simulink model "Buck_Converter_Model"  (R2020a)
settings: Solver=VariableStepAuto  StartTime=0.0  StopTime=0.4  RelTol=1e-3
libraries: powerlib x16, powerlib_meascontrol x2
settings Model: Creator=Ricardo Romero  LastModifiedBy=Ricardo Romero

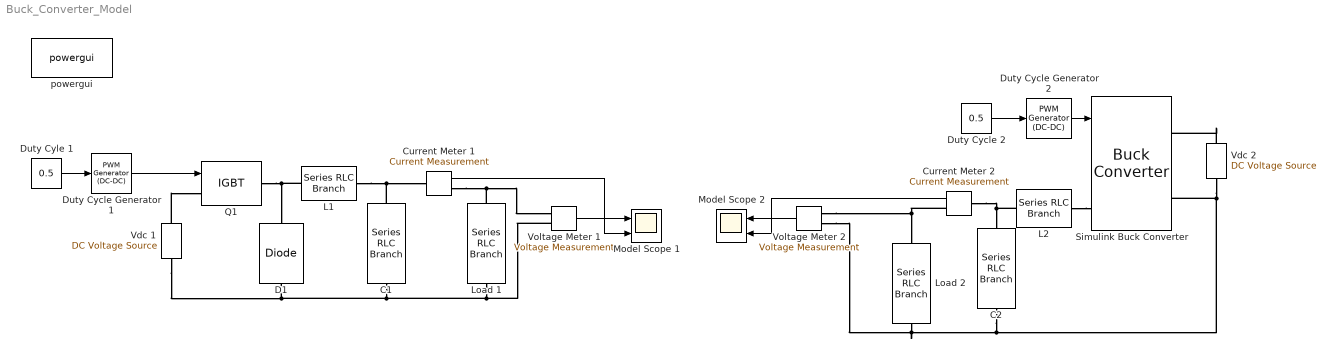
== system Buck_Converter_Model ==
  C1 : powerlib/Elements/Series RLC Branch  LConnTagsString=__new0  RConnTagsString=__new0  BranchType=C  Resistance=1  Inductance=1e-3  SetiL0=off  InitialCurrent=0  Capacitance=1e-3  Setx0=off  InitialVoltage=0  Measurements=None
  C2 : powerlib/Elements/Series RLC Branch  LConnTagsString=__new0  RConnTagsString=__new0  BranchType=C  Resistance=1  Inductance=1e-3  SetiL0=off  InitialCurrent=0  Capacitance=10e-3  Setx0=off  InitialVoltage=0  Measurements=None
  Current Meter 1 : powerlib/Measurements/Current Measurement  PhasorSimulation=off  OutputType=Complex  PSBequivalent=0
  Current Meter 2 : powerlib/Measurements/Current Measurement  PhasorSimulation=off  OutputType=Complex  PSBequivalent=0
  D1 : powerlib/Power Electronics/Diode  Ron=0.001  Lon=0  Vf=0.8  IC=0  UseSnubber=0  Rs=500  Cs=250e-9  Measurements=off
  Duty Cycle Generator 1 : powerlib_meascontrol/Pulse & Signal Generators/PWM Generator (DC-DC)  Fsw=5000  Ts=0
  Duty Cycle Generator 2 : powerlib_meascontrol/Pulse & Signal Generators/PWM Generator (DC-DC)  Fsw=5000  Ts=0
  Duty Cycle 2 : Constant  Value=0.5
  Duty Cyle 1 : Constant  Value=0.5
  L1 : powerlib/Elements/Series RLC Branch  LConnTagsString=__new0  RConnTagsString=__new0  BranchType=L  Resistance=1  Inductance=1e-3  SetiL0=off  InitialCurrent=0  Capacitance=1e-6  Setx0=off  InitialVoltage=0  Measurements=None
  L2 : powerlib/Elements/Series RLC Branch  LConnTagsString=__new0  RConnTagsString=__new0  BranchType=L  Resistance=1  Inductance=1e-3  SetiL0=off  InitialCurrent=0  Capacitance=1e-6  Setx0=off  InitialVoltage=0  Measurements=None
  Load 1 : powerlib/Elements/Series RLC Branch  LConnTagsString=__new0  RConnTagsString=__new0  BranchType=R  Resistance=10  Inductance=1e-3  SetiL0=off  InitialCurrent=0  Capacitance=1e-6  Setx0=off  InitialVoltage=0  Measurements=None
  Load 2 : powerlib/Elements/Series RLC Branch  LConnTagsString=__new0  RConnTagsString=__new0  BranchType=R  Resistance=10  Inductance=1e-3  SetiL0=off  InitialCurrent=0  Capacitance=1e-6  Setx0=off  InitialVoltage=0  Measurements=None
  Model Scope 1 : Scope  NumInputPorts=2
  Model Scope 2 : Scope  NumInputPorts=2
  Q1 : powerlib/Power Electronics/IGBT  Ron=0.001  Lon=0  Vf=1  Tf=1e-6  Tt=2e-6  IC=0  Rs=1e5  Cs=inf  Measurements=off
  Simulink Buck Converter : powerlib/Power Electronics/Buck Converter  ModelType=Switching devices  Ron=1e-3  Rs=1e6  Cs=inf  Vforward=[0,0]  Ron_Diode=1e-3  Rs_Diode=1e6  Cs_Diode=inf  Vf_Diode=1e-3  Rs_CurrentSource=inf
      settings: SourceProductBaseCode=PS
  Vdc 1 : powerlib/Electrical Sources/DC Voltage Source  Amplitude=10  Measurements=None
  Vdc 2 : powerlib/Electrical Sources/DC Voltage Source  Amplitude=10  Measurements=None
  Voltage Meter 1 : powerlib/Measurements/Voltage Measurement  PhasorSimulation=off  OutputType=Complex  PSBequivalent=0
  Voltage Meter 2 : powerlib/Measurements/Voltage Measurement  PhasorSimulation=off  OutputType=Complex  PSBequivalent=0
  powergui : powerlib/powergui  Priority=1  SimulationMode=Discrete  SampleTime=5e-6  frequency=60  Iterations=50  frequencyindice=0  Pbase=100e6  ErrMax=1e-4  UnitsV=kV  UnitsW=MW  buscounter=0  FunctionMessages=off  echomessages=off  EnableUseOfTLC=off  CurrentSourceSwitches=off  DisableSnubberDevices=off  DisableRonSwitches=off  DisableVfSwitches=off  DisplayEquations=off  AutomaticDiscreteSolvers=off  SolverType=Tustin/Backward Euler (TBE)  Interpol=off  ExternalGateDelay=off  methode=off  Ts=100  x0status=blocks  SPID=on  SwTol=0  HookPort=off  NonlinearTolerance=1e-4  nMaxIteration=100  ContinueOnMaxIteration=off  RestoreLinks=warning  ResistiveCurrentMeasurement=off  Frange=[0:2:500]  Ylog=off  Xlog=on  ShowGrid=off  save=off  variable=ZData  structure=0  ZoomFFT=off  StartTime=0.0  cycles=1  DisplayStyle=1  fundamental=60  FreqAxis=off  MaxFrequency=1000  frequencyindicesteady=1  RmsSteady=1  display=off
  wires:
  Voltage Meter 1/1 -> Model Scope 1/1
  Current Meter 1/1 -> Model Scope 1/2
  Duty Cyle 1/1 -> Duty Cycle Generator 1/1
  Duty Cycle Generator 1/1 -> Q1/1
  Duty Cycle 2/1 -> Duty Cycle Generator 2/1
  Duty Cycle Generator 2/1 -> Simulink Buck Converter/1
  Current Meter 2/1 -> Model Scope 2/2
  Voltage Meter 2/1 -> Model Scope 2/1
  connections:
  Load 1/LConn1 -- Current Meter 1/RConn1 -- Voltage Meter 1/LConn1
  Vdc 1/LConn1 -- Voltage Meter 1/LConn2 -- Load 1/RConn1 -- C1/RConn1 -- D1/LConn1
  C1/LConn1 -- Current Meter 1/LConn1 -- L1/RConn1
  Q1/RConn1 -- D1/RConn1 -- L1/LConn1
  Vdc 1/RConn1 -- Q1/LConn1
  L2/LConn1 -- Simulink Buck Converter/LConn1
  Vdc 2/RConn1 -- Simulink Buck Converter/RConn1
  Vdc 2/LConn1 -- Load 2/RConn1 -- Voltage Meter 2/LConn2 -- C2/RConn1 -- Simulink Buck Converter/RConn2
  L2/RConn1 -- Current Meter 2/LConn1 -- C2/LConn1
  Current Meter 2/RConn1 -- Load 2/LConn1 -- Voltage Meter 2/LConn1
